simulink model "ans5_65070121_155_168"  (R2024b)
settings: Solver=VariableStepAuto  StartTime=0.0  StopTime=10.0  RelTol=1e-3
libraries: commdigbbndpm3 x1, commrandsrc3 x1
settings Model: Creator=picha  LastModifiedBy=picha

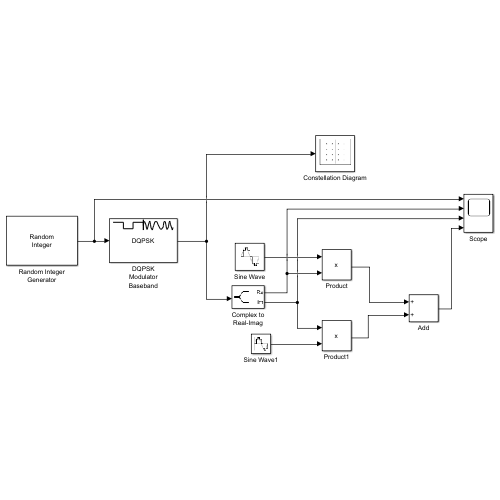
[thumbnail: Simulink's stored preview of the top-level diagram]
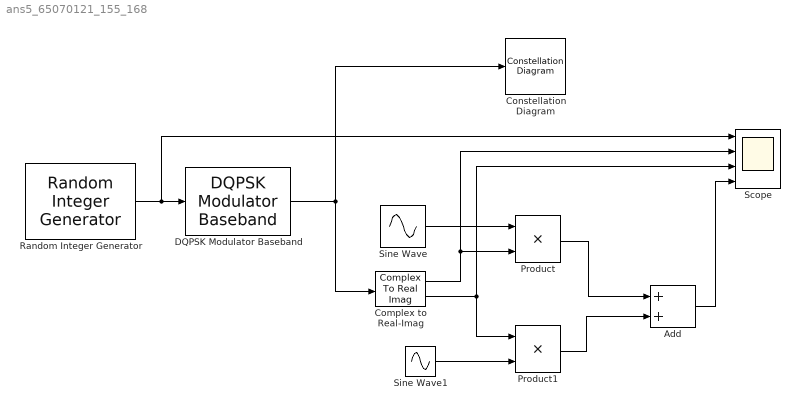
== system ans5_65070121_155_168 ==
  Add : Sum
  Complex to Real-Imag : ComplexToRealImag
  Constellation Diagram : ConstellationDiagram  WindowPosition=[885.000000,168.000000,600.000000,600.000000,]  Visible=on  ScopeFrameLocation=window
  DQPSK Modulator Baseband : commdigbbndpm3/DQPSK Modulator Baseband  InType=Integer  Enc=Gray  Ph=pi/4  outDtype=double
  Product : Product
  Product1 : Product
  Random Integer Generator : commrandsrc3/Random Integer Generator  SetSize=4  SeedSource=Auto  Seed=0  SampleTime=1  SamplesPerFrame=1  OutputDataType=double  SimulateUsing=Interpreted execution
  Scope : Scope  NumInputPorts=4
  Sine Wave : Sin  Frequency=4*pi  SampleTime=0.001
  Sine Wave1 : Sin  Frequency=4*pi  Phase=pi/2  SampleTime=0.001
  wires:
  Random Integer Generator/1 -> Scope/1, DQPSK Modulator Baseband/1
  DQPSK Modulator Baseband/1 -> Complex to Real-Imag/1, Constellation Diagram/1
  Sine Wave/1 -> Product/1
  Complex to Real-Imag/1 -> Product/2, Scope/2
  Complex to Real-Imag/2 -> Product1/1, Scope/3
  Sine Wave1/1 -> Product1/2
  Product/1 -> Add/1
  Product1/1 -> Add/2
  Add/1 -> Scope/4
